simulink model "Lab1"  (R2022b)
settings: Solver=VariableStepAuto  StartTime=0.0  StopTime=10.0  RelTol=1e-3
undefined symbols (not defined in the file): unicycle
libraries: simulink_extras x2
settings Model: Creator=Musta  LastModifiedBy=Musta

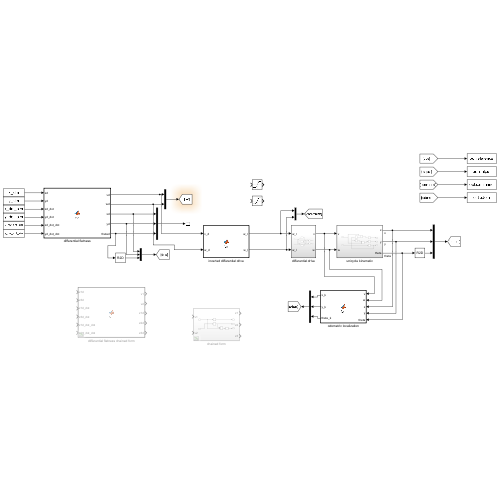
[thumbnail: Simulink's stored preview of the top-level diagram]
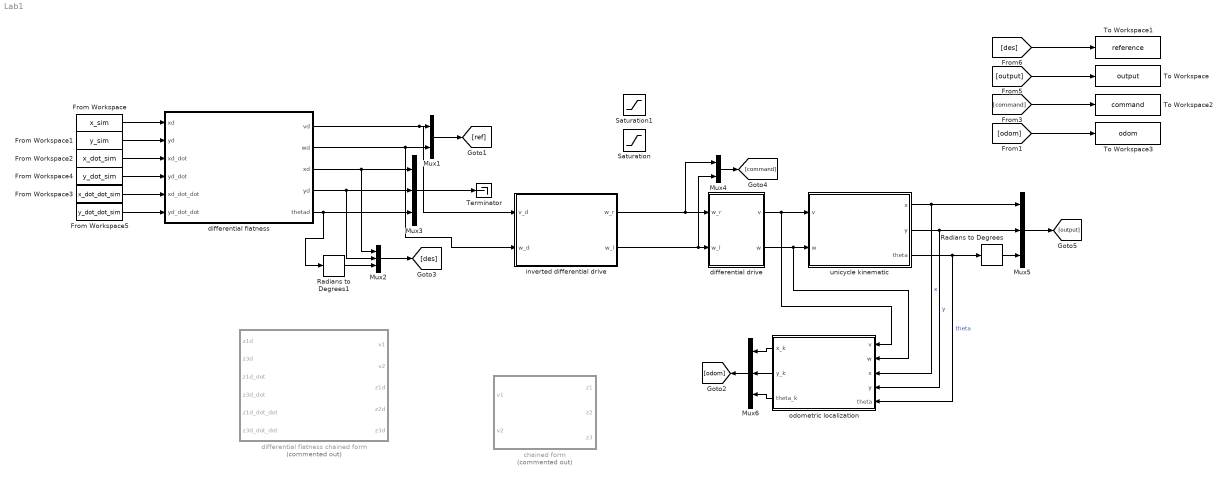
== system Lab1 ==
  From Workspace : FromWorkspace  VariableName=x_sim
  From Workspace1 : FromWorkspace  VariableName=y_sim
  From Workspace2 : FromWorkspace  VariableName=x_dot_sim
  From Workspace3 : FromWorkspace  VariableName=x_dot_dot_sim
  From Workspace4 : FromWorkspace  VariableName=y_dot_sim
  From Workspace5 : FromWorkspace  VariableName=y_dot_dot_sim
  Mux1 : Mux  Inputs=2
  Mux{2..3,5..6} (4 alike) : Mux  Inputs=3
  Mux4 : Mux  Inputs=2
  Radians to Degrees : simulink_extras/Transformations/Radians to Degrees
  Radians to Degrees1 : simulink_extras/Transformations/Radians to Degrees
  Saturation : Saturate  UpperLimit=unicycle.omegaWheelMax  LowerLimit=unicycle.omegaWheelMin
  Saturation1 : Saturate  UpperLimit=unicycle.omegaWheelMax  LowerLimit=unicycle.omegaWheelMin
  Terminator : Terminator
  To Workspace : ToWorkspace  VariableName=output  SaveFormat=Structure With Time  SampleTime=-1
  To Workspace1 : ToWorkspace  VariableName=reference  SaveFormat=Structure With Time  SampleTime=-1
  To Workspace2 : ToWorkspace  VariableName=command  SaveFormat=Structure With Time  SampleTime=-1
  To Workspace3 : ToWorkspace  VariableName=odom  SaveFormat=Structure With Time  SampleTime=-1
  chained form : Subsystem  Commented=on
  differential drive : Subsystem
  differential flatness : MATLAB Function  TreatAsAtomicUnit=on
  differential flatness chained form : MATLAB Function  Commented=on  TreatAsAtomicUnit=on
  inverted differential drive : MATLAB Function  TreatAsAtomicUnit=on
  odometric localization : MATLAB Function  TreatAsAtomicUnit=on
  unicycle kinematic : Subsystem
  wires:
  From Workspace5/1 -> differential flatness/6(yd_dot_dot)
  From Workspace4/1 -> differential flatness/4(yd_dot)
  Radians to Degrees/1 -> Mux5/3
  From Workspace3/1 -> differential flatness/5(xd_dot_dot)
  differential flatness/4(yd) -> Mux2/2, Mux3/2
  differential flatness/3(xd) -> Mux2/1, Mux3/1
  From Workspace1/1 -> differential flatness/2("yd ")
  differential flatness/5(thetad) -> Mux3/3, Radians to Degrees1/1
  From Workspace2/1 -> differential flatness/3(xd_dot)
  Mux5/1 -> [output]
  Mux1/1 -> [ref]
  differential flatness/2(wd) -> inverted differential drive/2(w_d), Mux1/2
  Radians to Degrees1/1 -> Mux2/3
  Mux3/1 -> Terminator/1
  unicycle kinematic/3(theta) -> odometric localization/5(theta), Radians to Degrees/1  "theta"
  From Workspace/1 -> differential flatness/1("xd ")
  [des] -> To Workspace1/1
  [command] -> To Workspace2/1
  [output] -> To Workspace/1
  differential flatness/1(vd) -> inverted differential drive/1(v_d), Mux1/1
  Mux2/1 -> [des]
  Mux4/1 -> [command]
  differential drive/1(v) -> odometric localization/1(v), unicycle kinematic/1(v)
  differential drive/2(w) -> odometric localization/2(w), unicycle kinematic/2(w)
  inverted differential drive/2(w_l) -> Mux4/2, differential drive/2(w_l)
  inverted differential drive/1(w_r) -> Mux4/1, differential drive/1(w_r)
  unicycle kinematic/1(x) -> odometric localization/3(x), Mux5/1  "x"
  unicycle kinematic/2(y) -> odometric localization/4(y), Mux5/2  "y"
  odometric localization/2(y_k) -> Mux6/2
  odometric localization/3(theta_k) -> Mux6/3
  odometric localization/1(x_k) -> Mux6/1
  Mux6/1 -> [odom]
  [odom] -> To Workspace3/1

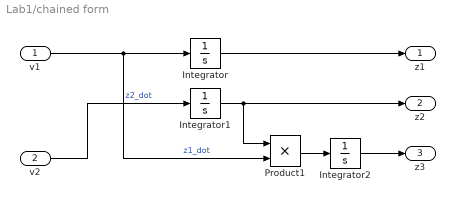
== system Lab1/chained form ==
  v1 : Inport
  v2 : Inport  Port=2
  Integrator : Integrator
  Integrator1 : Integrator
  Integrator2 : Integrator
  Product1 : Product
  z1 : Outport
  z2 : Outport  Port=2
  z3 : Outport  Port=3
  wires:
  Integrator2/1 -> z3/1
  Integrator1/1 -> Product1/1, z2/1
  v1/1 -> Product1/2, Integrator/1  "z1_dot"
  Integrator/1 -> z1/1
  v2/1 -> Integrator1/1  "z2_dot"
  Product1/1 -> Integrator2/1

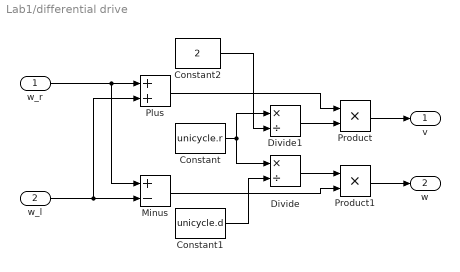
== system Lab1/differential drive ==
  w_r : Inport
  w_l : Inport  Port=2
  Constant : Constant  Value=unicycle.r
  Constant1 : Constant  Value=unicycle.d
  Constant2 : Constant  Value=2
  Divide : Product  Inputs=*/
  Divide1 : Product  Inputs=*/
  Minus : Sum  Inputs=+-
  Plus : Sum
  Product : Product
  Product1 : Product
  v : Outport
  w : Outport  Port=2
  wires:
  w_r/1 -> Minus/1, Plus/1
  w_l/1 -> Minus/2, Plus/2
  Product/1 -> v/1
  Product1/1 -> w/1
  Constant/1 -> Divide/1, Divide1/1
  Constant2/1 -> Divide1/2
  Divide1/1 -> Product/2
  Plus/1 -> Product/1
  Constant1/1 -> Divide/2
  Minus/1 -> Product1/2
  Divide/1 -> Product1/1

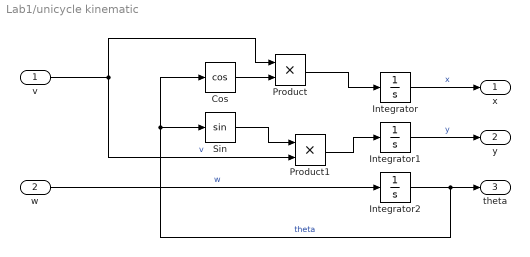
== system Lab1/unicycle kinematic ==
  v : Inport
  w : Inport  Port=2
  Cos : Trigonometry  Operator=cos
  Integrator : Integrator  InitialCondition=unicycle.ic.x
  Integrator1 : Integrator  InitialCondition=unicycle.ic.y
  Integrator2 : Integrator  InitialCondition=unicycle.ic.theta
  Product : Product
  Product1 : Product
  Sin : Trigonometry
  x : Outport
  y : Outport  Port=2
  theta : Outport  Port=3
  wires:
  w/1 -> Integrator2/1  "w"
  Product/1 -> Integrator/1
  v/1 -> Product/1, Product1/2  "v"
  Cos/1 -> Product/2
  Integrator1/1 -> y/1  "y"
  Integrator/1 -> x/1  "x"
  Integrator2/1 -> Cos/1, Sin/1, theta/1  "theta"
  Product1/1 -> Integrator1/1
  Sin/1 -> Product1/1

== matlab function Lab1/inverted differential drive ==
  data: v_d input; w_r output; w_d input; w_l output
function [w_r, w_l] = fcn(v_d, w_d)

    %#codegen
    coder.extrinsic('evalin')
    d = 0;                  % Needed in order to set variable class correctly
    r = 0;                  % Needed in order to set variable class correctly
    d = evalin('base','unicycle.d'); % Read value from workspace
    r = evalin('base','unicycle.r'); % Read value from workspace

    w_r = ((2 * v_d) + (w_d * d)) / (2 * r);
    w_l = ((2 * v_d) - (w_d * d)) / (2 * r);

end

== matlab function Lab1/differential flatness ==
  data: xd input; vd output; yd input; xd_dot input; yd_dot input; xd_dot_dot input; yd_dot_dot input; wd output; xd output; yd output; thetad output
function [vd, wd, xd, yd, thetad] = fcn(xd, yd, xd_dot, yd_dot, xd_dot_dot, yd_dot_dot)
    
    vd = sqrt(xd_dot.^2 + yd_dot.^2);
    wd = (xd_dot.*yd_dot_dot - xd_dot_dot.*yd_dot) / (xd_dot.^2 + yd_dot.^2);
    % thetad = atan2(yd_dot, xd_dot);
    thetad = mod(atan2(yd_dot,xd_dot), 2*pi);

    xd = xd;
    yd = yd;

end

== matlab function Lab1/differential flatness chained form ==
  data: z1d input; v1 output; z3d input; z1d_dot input; z3d_dot input; z1d_dot_dot input; z3d_dot_dot input; v2 output; z1d output; z2d output; z3d output
function [v1, v2, z1d, z2d, z3d] = fcn(z1d, z3d, z1d_dot, z3d_dot, z1d_dot_dot, z3d_dot_dot)
    
    v1 = z1d_dot;
    v2 = (-z1d_dot_dot.*z3d_dot - z3d_dot_dot.*z1d_dot) / (z1d_dot^2);

    z1d = z1d;
    z2d = z3d_dot / z1d_dot;
    z3d = z3d;

end

== matlab function Lab1/odometric localization ==
  data: v input; x_k output; w input; y_k output; x input; y input; theta input; theta_k output
function [x_k, y_k, theta_k] = fcn(v, w, x, y, theta)

    %#codegen
    coder.extrinsic('evalin')
    Ts = 0;                  % Needed in order to set variable class correctly
    Ts = evalin('base','unicycle.Ts'); % Read value from workspace

    x_k = x + v*Ts*cos(theta + (w*Ts)/2);
    y_k = y + v*Ts*sin(theta + (w*Ts)/2);
    theta_k = theta + w*Ts;

end
